simulink model "Pendulum_Nonlinear_System"  (R2019a)
settings: Solver=ode45  StartTime=0.0  StopTime=T_sample*T_sim  RelTol=1e-3
values from neighbouring files (symbols this model uses):
  b = 1/1000    (= 0.001)    [MPC_Project_2021_Eyuboglu_main_code.m]    (also in MPC_Project_Pendulum_2021.m)
  g = 9.81    [MPC_Project_2021_Eyuboglu_main_code.m]    (also in MPC_Project_Pendulum_2021.m)
  J = m*l^2    (= 0.0007)    [MPC_Project_2021_Eyuboglu_main_code.m]    (also in MPC_Project_Pendulum_2021.m)
  k = 6/100    (= 0.06)    [MPC_Project_2021_Eyuboglu_main_code.m]    (also in MPC_Project_Pendulum_2021.m)
  l = 1/10    (= 0.1)    [MPC_Project_2021_Eyuboglu_main_code.m]    (also in MPC_Project_Pendulum_2021.m)
  L = 1/1000    (= 0.001)    [MPC_Project_2021_Eyuboglu_main_code.m]    (also in MPC_Project_Pendulum_2021.m; getWLc_TS.m = Mcal*Gamma+Ecal)
  m = 7/100    (= 0.07)    [MPC_Project_2021_Eyuboglu_main_code.m]    (also in MPC_Project_Pendulum_2021.m)
  R = 1    [MPC_Project_2021_Eyuboglu_main_code.m]    (also in MPC_Project_Pendulum_2021.m)
  T_sample = 0.004    [MPC_Project_2021_Eyuboglu_main_code.m]    (also in MPC_Project_Pendulum_2021.m)
  u_input = u_mpc(i)    [MPC_Project_2021_Eyuboglu_main_code.m]    (also in MPC_Project_Pendulum_2021.m = 0)
  x1_0 = x(1,i)    [MPC_Project_2021_Eyuboglu_main_code.m]    (also in MPC_Project_Pendulum_2021.m = 1e-05)
  x2_0 = x(2,i)    [MPC_Project_2021_Eyuboglu_main_code.m]    (also in MPC_Project_Pendulum_2021.m = 0)
  x3_0 = x(3,i)    [MPC_Project_2021_Eyuboglu_main_code.m]    (also in MPC_Project_Pendulum_2021.m = 0)
settings Model: Creator=20205236  LastModifiedBy=20205236
settings DataIOCC: ReturnWorkspaceOutputs=off

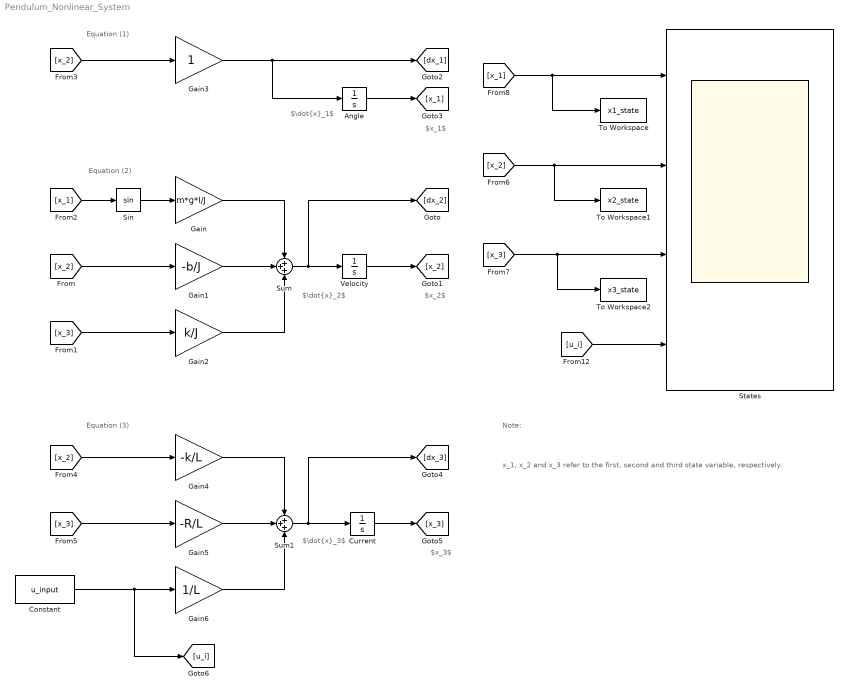
== system Pendulum_Nonlinear_System ==
  note: x_1, x_2 and x_3 refer to the first, second and third state variable, respectively.
  note: $x_2$
  note: $x_1$
  note: Equation (1)
  note: Equation (3)
  note: Equation (2)
  note: $x_3$
  note: $\dot{x}_3$
  note: $\dot{x}_2$
  note: $\dot{x}_1$
  note: Note:
  Angle : Integrator  InitialCondition=x1_0
  Constant : Constant  Value=u_input
  Current : Integrator  InitialCondition=x3_0
  Gain : Gain  Gain=m*g*l/J
  Gain1 : Gain  Gain=-b/J
  Gain2 : Gain  Gain=k/J
  Gain3 : Gain
  Gain4 : Gain  Gain=-k/L
  Gain5 : Gain  Gain=-R/L
  Gain6 : Gain  Gain=1/L
  Sin : Trigonometry
  States : Scope  NumInputPorts=4
  Sum : Sum  Inputs=+++
  Sum1 : Sum  Inputs=+++
  To Workspace : ToWorkspace  VariableName=x1_state  SampleTime=T_sample
  To Workspace1 : ToWorkspace  VariableName=x2_state  SampleTime=T_sample
  To Workspace2 : ToWorkspace  VariableName=x3_state  SampleTime=T_sample
  Velocity : Integrator  InitialCondition=x2_0
  wires:
  Sin/1 -> Gain/1
  Gain1/1 -> Sum/2
  Gain2/1 -> Sum/3
  Gain/1 -> Sum/1
  Sum/1 -> Velocity/1, [dx_2]
  Velocity/1 -> [x_2]
  [x_2] -> Gain1/1
  [x_3] -> Gain2/1
  [x_1] -> Sin/1
  [x_2] -> Gain3/1
  Gain3/1 -> Angle/1, [dx_1]
  Angle/1 -> [x_1]
  [x_2] -> Gain4/1
  Gain4/1 -> Sum1/1
  Constant/1 -> [u_i], Gain6/1
  Gain5/1 -> Sum1/2
  [x_3] -> Gain5/1
  Current/1 -> [x_3]
  Gain6/1 -> Sum1/3
  Sum1/1 -> Current/1, [dx_3]
  [x_1] -> To Workspace/1, States/1
  [x_3] -> To Workspace2/1, States/3
  [x_2] -> To Workspace1/1, States/2
  [u_i] -> States/4
